simulink model "kurwa_dziala"  (R2022b)
settings: Solver=VariableStepAuto  StartTime=0.0  StopTime=300  RelTol=1e-3
undefined symbols (not defined in the file): alfa_1, gravity_acceleration, i, Malpha, Malphadot, MdeltaE, Mq, Mtalpha, Mtu, Mu, o, Vp1, Xalpha, XdeltaE, Xtu, Xu, Zalpha, Zalphadot, ZdeltaE, Zq, Zu
libraries: simulink_extras x3
settings Model: Creator=48519  LastModifiedBy=48519

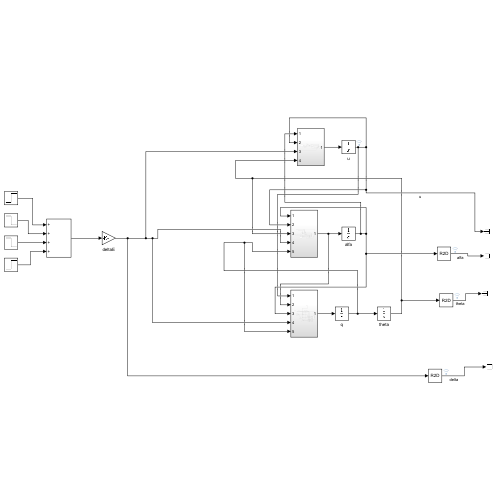
[thumbnail: Simulink's stored preview of the top-level diagram]
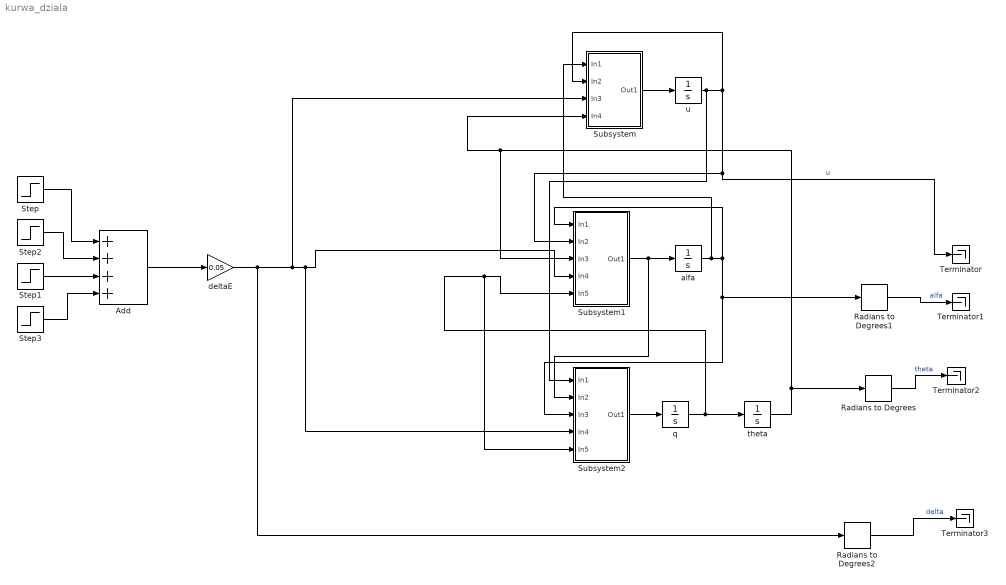
== system kurwa_dziala ==
  Add : Sum  Inputs=++++
  Radians to Degrees : simulink_extras/Transformations/Radians to Degrees
  Radians to Degrees1 : simulink_extras/Transformations/Radians to Degrees
  Radians to Degrees2 : simulink_extras/Transformations/Radians to Degrees
  Step : Step  Time=2  SampleTime=0
  Step1 : Step  Time=62  After=-1  SampleTime=0
  Step2 : Step  Time=4  After=-1  SampleTime=0
  Step3 : Step  Time=64  SampleTime=0
  Subsystem : Subsystem
  Subsystem1 : Subsystem
  Subsystem2 : Subsystem
  Terminator{,1..3} (4 alike) : Terminator
  alfa : Integrator
  deltaE : Gain  Gain=0.05
  q : Integrator
  theta : Integrator
  u : Integrator
  wires:
  Step/1 -> Add/1
  Step2/1 -> Add/2
  Step1/1 -> Add/3
  Step3/1 -> Add/4
  Add/1 -> deltaE/1
  alfa/1 -> Subsystem1/1(In1), Radians to Degrees1/1, Subsystem2/3(In3), Subsystem/1(In1)
  u/1 -> Subsystem/2(In2), Terminator/1, Subsystem1/2(In2), Subsystem2/1(In1)  "u"
  deltaE/1 -> Radians to Degrees2/1, Subsystem2/4(In4), Subsystem1/4(In4), Subsystem/3(In3)
  theta/1 -> Radians to Degrees/1, Subsystem/4(In4), Subsystem1/3(In3)
  Subsystem/1(Out1) -> u/1
  q/1 -> Subsystem2/5(In5), Subsystem1/5(In5), theta/1
  Subsystem1/1(Out1) -> Subsystem2/2(In2), alfa/1
  Subsystem2/1(Out1) -> q/1
  Radians to Degrees/1 -> Terminator2/1  "theta"
  Radians to Degrees1/1 -> Terminator1/1  "alfa"
  Radians to Degrees2/1 -> Terminator3/1  "delta"

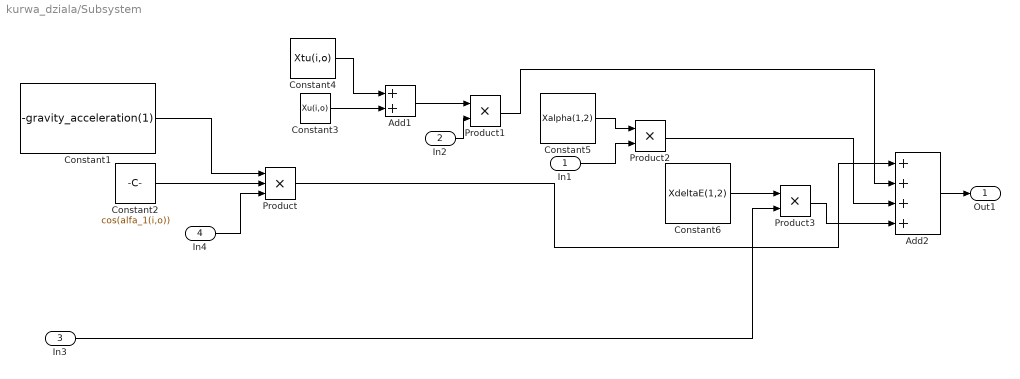
== system kurwa_dziala/Subsystem ==
  In1 : Inport
  In2 : Inport  Port=2
  In3 : Inport  Port=3
  In4 : Inport  Port=4
  Add1 : Sum
  Add2 : Sum  Inputs=++++
  Constant1 : Constant  Value=-gravity_acceleration(1)
  Constant2 : Constant  Value=cos(alfa_1(i,o))
  Constant3 : Constant  Value=Xu(i,o)
  Constant4 : Constant  Value=Xtu(i,o)
  Constant5 : Constant  Value=Xalpha(1,2)
  Constant6 : Constant  Value=XdeltaE(1,2)
  Product : Product  Inputs=3
  Product1 : Product
  Product2 : Product
  Product3 : Product
  Out1 : Outport
  wires:
  Constant4/1 -> Add1/1
  Add1/1 -> Product1/1
  Constant3/1 -> Add1/2
  Product3/1 -> Add2/4
  Product/1 -> Add2/1
  Constant1/1 -> Product/1
  Add2/1 -> Out1/1
  Constant2/1 -> Product/2
  Product2/1 -> Add2/3
  Product1/1 -> Add2/2
  Constant5/1 -> Product2/1
  Constant6/1 -> Product3/1
  In2/1 -> Product1/2
  In4/1 -> Product/3
  In1/1 -> Product2/2
  In3/1 -> Product3/2

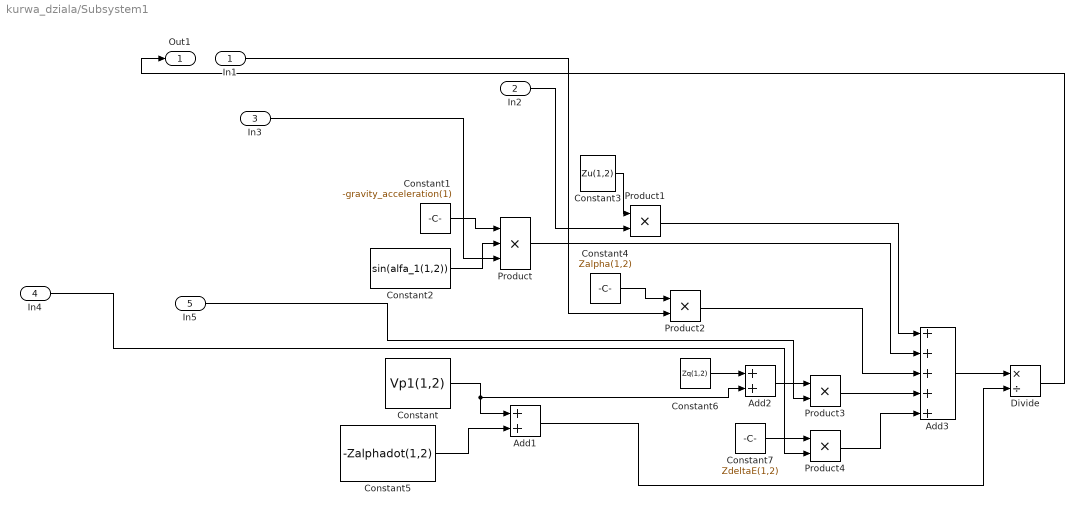
== system kurwa_dziala/Subsystem1 ==
  In1 : Inport
  In2 : Inport  Port=2
  In3 : Inport  Port=3
  In4 : Inport  Port=4
  In5 : Inport  Port=5
  Add1 : Sum
  Add2 : Sum
  Add3 : Sum  Inputs=+++++
  Constant : Constant  Value=Vp1(1,2)
  Constant1 : Constant  Value=-gravity_acceleration(1)
  Constant2 : Constant  Value=sin(alfa_1(1,2))
  Constant3 : Constant  Value=Zu(1,2)
  Constant4 : Constant  Value=Zalpha(1,2)
  Constant5 : Constant  Value=-Zalphadot(1,2)
  Constant6 : Constant  Value=Zq(1,2)
  Constant7 : Constant  Value=ZdeltaE(1,2)
  Divide : Product  Inputs=*/
  Product : Product  Inputs=3
  Product{1..4} (4 alike) : Product
  Out1 : Outport
  wires:
  Constant7/1 -> Product4/1
  Add2/1 -> Product3/1
  Constant5/1 -> Add1/2
  Constant2/1 -> Product/2
  Constant/1 -> Add2/2, Add1/1
  Constant4/1 -> Product2/1
  Add3/1 -> Divide/1
  Constant6/1 -> Add2/1
  Product4/1 -> Add3/5
  In3/1 -> Product/3
  Product/1 -> Add3/2
  Product2/1 -> Add3/3
  Constant1/1 -> Product/1
  In5/1 -> Product3/2
  Product3/1 -> Add3/4
  Constant3/1 -> Product1/1
  Product1/1 -> Add3/1
  Add1/1 -> Divide/2
  In1/1 -> Product2/2
  In4/1 -> Product4/2
  In2/1 -> Product1/2
  Divide/1 -> Out1/1

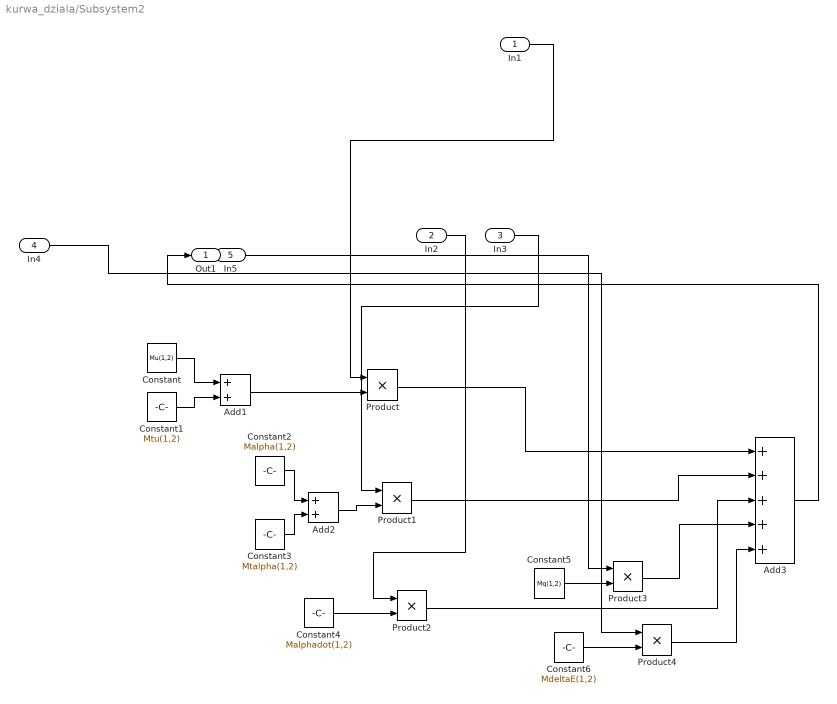
== system kurwa_dziala/Subsystem2 ==
  In1 : Inport
  In2 : Inport  Port=2
  In3 : Inport  Port=3
  In4 : Inport  Port=4
  In5 : Inport  Port=5
  Add1 : Sum
  Add2 : Sum
  Add3 : Sum  Inputs=+++++
  Constant : Constant  Value=Mu(1,2)
  Constant1 : Constant  Value=Mtu(1,2)
  Constant2 : Constant  Value=Malpha(1,2)
  Constant3 : Constant  Value=Mtalpha(1,2)
  Constant4 : Constant  Value=Malphadot(1,2)
  Constant5 : Constant  Value=Mq(1,2)
  Constant6 : Constant  Value=MdeltaE(1,2)
  Product{,1..4} (5 alike) : Product
  Out1 : Outport
  wires:
  Constant1/1 -> Add1/2
  Constant6/1 -> Product4/2
  Constant2/1 -> Add2/1
  Product3/1 -> Add3/4
  Add2/1 -> Product1/2
  Product2/1 -> Add3/3
  Product1/1 -> Add3/2
  Product4/1 -> Add3/5
  Constant4/1 -> Product2/2
  Constant/1 -> Add1/1
  Add1/1 -> Product/2
  In5/1 -> Product3/1
  In3/1 -> Product1/1
  Product/1 -> Add3/1
  Add3/1 -> Out1/1
  Constant3/1 -> Add2/2
  Constant5/1 -> Product3/2
  In2/1 -> Product2/1
  In4/1 -> Product4/1
  In1/1 -> Product/1
